simulink model "robot_turn_2"  (R2023a)
settings: Solver=FixedStepDiscrete  StartTime=0.0  StopTime=100  FixedStep=0.01  RelTol=1e-3
libraries: mobileRoboticsTrainingLib x3
settings Model: NumberOfSteps=10  SnapshotBufferSize=100  Creator=Boitumelo  LastModifiedBy=thuto
settings DebuggingCC: UnconnectedInputMsg=warning  UnconnectedOutputMsg=warning  UnconnectedLineMsg=warning
settings ModelReferenceCC: EnableRefExpFcnMdlSchedulingChecks=on
settings RTWCC: DLArmComputeVersion=19.05

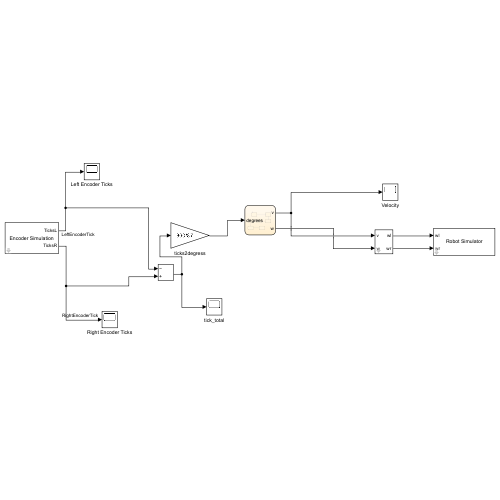
[thumbnail: Simulink's stored preview of the top-level diagram]
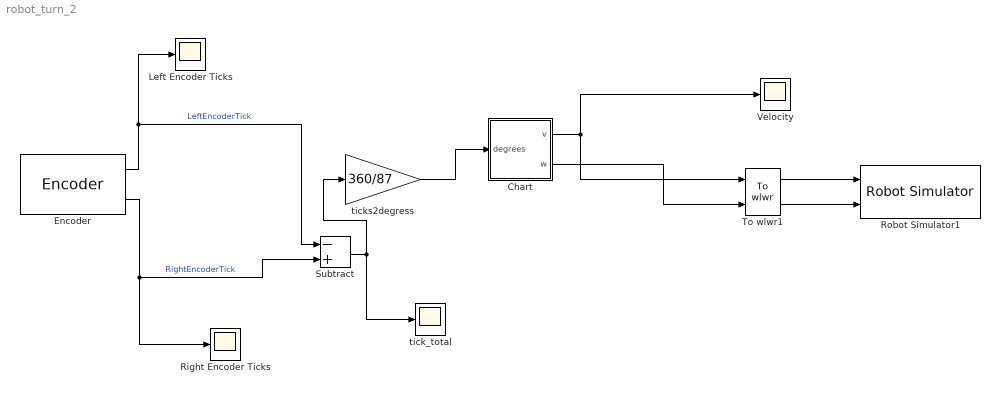
== system robot_turn_2 ==
  Chart : Stateflow chart  TreatAsAtomicUnit=on
  Encoder : mobileRoboticsTrainingLib/Encoder  axleLength=axleLength  wheelR=wheelR  ticksPerRot=ticksPerRot
      settings: SourceProductName=Mobile Robotics Training Library
  Left Encoder Ticks : Scope
  Right Encoder Ticks : Scope
  Robot Simulator1 : mobileRoboticsTrainingLib/Robot Simulator  Priority=99  mapVar=mapForSim  startX=0.82657  startY=1.0031  startTheta=0  axleLength=axleLength  wheelR=wheelR
  Subtract : Sum  Inputs=-+
  To wlwr1 : mobileRoboticsTrainingLib/To wlwr  axleLength=0.1  wheelR=0.05
  Velocity : Scope
  tick_total : Scope
  ticks2degress : Gain  Gain=360/87
  wires:
  Encoder/1 -> Left Encoder Ticks/1, Subtract/1  "LeftEncoderTick"
  Encoder/2 -> Subtract/2, Right Encoder Ticks/1  "RightEncoderTick"
  Chart/1(v) -> Velocity/1, To wlwr1/1
  To wlwr1/1 -> Robot Simulator1/1
  To wlwr1/2 -> Robot Simulator1/2
  Chart/2(w) -> To wlwr1/2
  Subtract/1 -> tick_total/1, ticks2degress/1
  ticks2degress/1 -> Chart/1(degrees)

== stateflow chart robot_turn_2/Chart ==
  state startTurn90
    entry: v=0
    w=1
  state resetPos1
    entry: v=0
    w=-1
  state startTurn270
    entry: v=0
    w=1
  state resetPos2
    entry: v=0
    w=-1
  state startTurn180
    entry: v=0
    w=1
  state resetPos3
    entry: v=0
    w=-1
  state stop
    entry: v=0
    w=0
  (default) -> startTurn90
  startTurn90 -> resetPos1 : [degrees>= 90]
  resetPos1 -> startTurn180 : [degrees < 0]
  resetPos2 -> startTurn270 : [degrees < 0]
  startTurn180 -> resetPos2 : [degrees>=180]
  startTurn270 -> resetPos3 : [degrees>=270]
  resetPos3 -> stop : [degrees < 0]
  data: v output; w output; degrees input
